simulink model "towing_project"  (Simulink 10.1)
settings: Solver=ode4  StartTime=0.0  StopTime=800  FixedStep=1  RelTol=1e-3  EnableMultiTasking=on
PreLoadFcn:
  | load('Initialization_data.mat');
undefined symbols (not defined in the file): D, D1, M, M1, Ma, Ma1, magnitude, p00, p10, p20, p30, p40
libraries: simulink x10, simulink_extras x4
(part 2 of 2)

== system towing_project/local DP1/Tug DP controller/[-inf inf] to [-pi pi]2 ==
  note: r
  note: x
  x [-inf inf] : Inport
  Constant : Constant  Value=2*pi
  Gain : Gain  Gain=pi  SaturateOnIntegerOverflow=on  OutDataTypeStr=Inherit: Same as input  ParamDataTypeStr=Inherit: Same as input
  Math Function : Math  Operator=rem  SignedPower=on  SaturateOnIntegerOverflow=on
  Saturation : Saturate  UpperLimit=1e10  LowerLimit=-1e10
  Sign : Signum
  Sum : Sum  Inputs=|+-  SaturateOnIntegerOverflow=on
  Sum1 : Sum  Inputs=|++  SaturateOnIntegerOverflow=on
  y [-pi pi] : Outport
  wires:
  Saturation/1 -> Sign/1, Sum1/1
  Sum/1 -> y [-pi pi]/1
  Math Function/1 -> Sum/1
  Constant/1 -> Math Function/2
  Sum1/1 -> Math Function/1
  Gain/1 -> Sum1/2, Sum/2
  Sign/1 -> Gain/1
  x [-inf inf]/1 -> Saturation/1

== system towing_project/local DP2/Tug/Coriolis and centripetal forces ==
  nu : Inport
  Mux : Mux  Inputs=3
  Selector1 : Selector  InputPortWidth=3  IndexOptions=Index vector (dialog)  Indices=[1 ]  OutputSizes=1
  Selector2 : Selector  InputPortWidth=3  IndexOptions=Index vector (dialog)  Indices=[2]  OutputSizes=1
  Selector3 : Selector  InputPortWidth=3  IndexOptions=Index vector (dialog)  Indices=[3]  OutputSizes=1
  Subsystem : Subsystem
  Subsystem1 : Subsystem
  Subsystem2 : Subsystem
  Output : Outport
  wires:
  nu/1 -> Selector1/1, Selector2/1, Selector3/1
  Selector2/1 -> Subsystem/1(v), Subsystem2/2(v)  "v"
  Selector3/1 -> Subsystem/2(r), Subsystem1/2(r), Subsystem2/3(r)  "r"
  Selector1/1 -> Subsystem1/1(u), Subsystem2/1(u)  "u"
  Subsystem/1(x direction) -> Mux/1
  Subsystem1/1(y direction) -> Mux/2
  Subsystem2/1(yaw direction) -> Mux/3
  Mux/1 -> Output/1

== system towing_project/local DP2/Tug/In Case of singularity ==
  input : Inport
  Compare To Constant : simulink/Logic and Bit Operations/Compare To Constant  relop=>=  const=1e8  OutDataTypeStr=boolean
  Stop Simulation : Stop
  output : Outport
  wires:
  input/1 -> output/1, Compare To Constant/1
  Compare To Constant/1 -> Stop Simulation/1

== system towing_project/local DP2/Tug/In Case of singularity1 ==
  input : Inport
  Compare To Constant : simulink/Logic and Bit Operations/Compare To Constant  relop=>=  const=1e10  OutDataTypeStr=boolean
  Stop Simulation : Stop
  output : Outport
  wires:
  input/1 -> output/1, Compare To Constant/1
  Compare To Constant/1 -> Stop Simulation/1

== system towing_project/local DP2/Tug/Rotation matrix in yaw ==
  psi : Inport
  nu : Inport  Port=2
  Fcn : Fcn  Expr=cos(u(1))*u(2)-sin(u(1))*u(3)
  Fcn1 : Fcn  Expr=sin(u(1))*u(2)+cos(u(1))*u(3)
  Fcn2 : Fcn  Expr=u(4)
  Mux : Mux  Inputs=2
  Mux1 : Mux  Inputs=3
  R*nu : Outport
  wires:
  Mux1/1 -> R*nu/1  "eta_dot"
  Mux/1 -> Fcn/1, Fcn1/1, Fcn2/1
  psi/1 -> Mux/1
  nu/1 -> Mux/2
  Fcn1/1 -> Mux1/2  "y_dot"
  Fcn/1 -> Mux1/1  "x_dot"
  Fcn2/1 -> Mux1/3  "psi_dot"

== system towing_project/local DP2/Tug/[-inf inf] to [-pi pi]1 ==
  note: x
  note: r
  x [-inf inf] : Inport
  Constant : Constant  Value=2*pi
  Gain : Gain  Gain=pi  SaturateOnIntegerOverflow=on  OutDataTypeStr=Inherit: Same as input  ParamDataTypeStr=Inherit: Same as input
  Math Function : Math  Operator=rem  SignedPower=on  SaturateOnIntegerOverflow=on
  Saturation : Saturate  UpperLimit=1e10  LowerLimit=-1e10
  Sign : Signum
  Sum : Sum  Inputs=|+-  SaturateOnIntegerOverflow=on
  Sum1 : Sum  Inputs=|++  SaturateOnIntegerOverflow=on
  y [-pi pi] : Outport
  wires:
  x [-inf inf]/1 -> Saturation/1
  Sign/1 -> Gain/1
  Gain/1 -> Sum/2, Sum1/2
  Sum1/1 -> Math Function/1
  Constant/1 -> Math Function/2
  Math Function/1 -> Sum/1
  Sum/1 -> y [-pi pi]/1
  Saturation/1 -> Sum1/1, Sign/1

== system towing_project/local DP2/Tug DP controller/Transposed rotation  matrix in yaw ==
  psi : Inport
  V : Inport  Port=2
  Mux : Mux  Inputs=2
  Mux1 : Mux  Inputs=3
  Row1 : Fcn  Expr=cos(u(1))*u(2)+sin(u(1))*u(3)
  Row2 : Fcn  Expr=-sin(u(1))*u(2)+cos(u(1))*u(3)
  Row3 : Fcn  Expr=u(4)
  Out1 : Outport
  wires:
  Mux/1 -> Row3/1, Row2/1, Row1/1
  Row1/1 -> Mux1/1
  Row2/1 -> Mux1/2
  Row3/1 -> Mux1/3
  Mux1/1 -> Out1/1
  psi/1 -> Mux/1
  V/1 -> Mux/2

== system towing_project/local DP2/Tug DP controller/[-inf inf] to [-pi pi]1 ==
  note: x
  note: r
  x [-inf inf] : Inport
  Constant : Constant  Value=2*pi
  Gain : Gain  Gain=pi  SaturateOnIntegerOverflow=on  OutDataTypeStr=Inherit: Same as input  ParamDataTypeStr=Inherit: Same as input
  Math Function : Math  Operator=rem  SignedPower=on  SaturateOnIntegerOverflow=on
  Saturation : Saturate  UpperLimit=1e10  LowerLimit=-1e10
  Sign : Signum
  Sum : Sum  Inputs=|+-  SaturateOnIntegerOverflow=on
  Sum1 : Sum  Inputs=|++  SaturateOnIntegerOverflow=on
  y [-pi pi] : Outport
  wires:
  x [-inf inf]/1 -> Saturation/1
  Sign/1 -> Gain/1
  Gain/1 -> Sum/2, Sum1/2
  Sum1/1 -> Math Function/1
  Constant/1 -> Math Function/2
  Math Function/1 -> Sum/1
  Sum/1 -> y [-pi pi]/1
  Saturation/1 -> Sum1/1, Sign/1

== system towing_project/local DP2/Tug DP controller/[-inf inf] to [-pi pi]2 ==
  note: r
  note: x
  x [-inf inf] : Inport
  Constant : Constant  Value=2*pi
  Gain : Gain  Gain=pi  SaturateOnIntegerOverflow=on  OutDataTypeStr=Inherit: Same as input  ParamDataTypeStr=Inherit: Same as input
  Math Function : Math  Operator=rem  SignedPower=on  SaturateOnIntegerOverflow=on
  Saturation : Saturate  UpperLimit=1e10  LowerLimit=-1e10
  Sign : Signum
  Sum : Sum  Inputs=|+-  SaturateOnIntegerOverflow=on
  Sum1 : Sum  Inputs=|++  SaturateOnIntegerOverflow=on
  y [-pi pi] : Outport
  wires:
  Saturation/1 -> Sign/1, Sum1/1
  Sum/1 -> y [-pi pi]/1
  Math Function/1 -> Sum/1
  Constant/1 -> Math Function/2
  Sum1/1 -> Math Function/1
  Gain/1 -> Sum1/2, Sum/2
  Sign/1 -> Gain/1
  x [-inf inf]/1 -> Saturation/1

== system towing_project/local DP3/Tug/Coriolis and centripetal forces ==
  nu : Inport
  Mux : Mux  Inputs=3
  Selector1 : Selector  InputPortWidth=3  IndexOptions=Index vector (dialog)  Indices=[1 ]  OutputSizes=1
  Selector2 : Selector  InputPortWidth=3  IndexOptions=Index vector (dialog)  Indices=[2]  OutputSizes=1
  Selector3 : Selector  InputPortWidth=3  IndexOptions=Index vector (dialog)  Indices=[3]  OutputSizes=1
  Subsystem : Subsystem
  Subsystem1 : Subsystem
  Subsystem2 : Subsystem
  Output : Outport
  wires:
  nu/1 -> Selector1/1, Selector2/1, Selector3/1
  Selector2/1 -> Subsystem/1(v), Subsystem2/2(v)  "v"
  Selector3/1 -> Subsystem/2(r), Subsystem1/2(r), Subsystem2/3(r)  "r"
  Selector1/1 -> Subsystem1/1(u), Subsystem2/1(u)  "u"
  Subsystem/1(x direction) -> Mux/1
  Subsystem1/1(y direction) -> Mux/2
  Subsystem2/1(yaw direction) -> Mux/3
  Mux/1 -> Output/1

== system towing_project/local DP3/Tug/In Case of singularity ==
  input : Inport
  Compare To Constant : simulink/Logic and Bit Operations/Compare To Constant  relop=>=  const=1e8  OutDataTypeStr=boolean
  Stop Simulation : Stop
  output : Outport
  wires:
  input/1 -> output/1, Compare To Constant/1
  Compare To Constant/1 -> Stop Simulation/1

== system towing_project/local DP3/Tug/In Case of singularity1 ==
  input : Inport
  Compare To Constant : simulink/Logic and Bit Operations/Compare To Constant  relop=>=  const=1e10  OutDataTypeStr=boolean
  Stop Simulation : Stop
  output : Outport
  wires:
  input/1 -> output/1, Compare To Constant/1
  Compare To Constant/1 -> Stop Simulation/1

== system towing_project/local DP3/Tug/Rotation matrix in yaw ==
  psi : Inport
  nu : Inport  Port=2
  Fcn : Fcn  Expr=cos(u(1))*u(2)-sin(u(1))*u(3)
  Fcn1 : Fcn  Expr=sin(u(1))*u(2)+cos(u(1))*u(3)
  Fcn2 : Fcn  Expr=u(4)
  Mux : Mux  Inputs=2
  Mux1 : Mux  Inputs=3
  R*nu : Outport
  wires:
  Mux1/1 -> R*nu/1  "eta_dot"
  Mux/1 -> Fcn/1, Fcn1/1, Fcn2/1
  psi/1 -> Mux/1
  nu/1 -> Mux/2
  Fcn1/1 -> Mux1/2  "y_dot"
  Fcn/1 -> Mux1/1  "x_dot"
  Fcn2/1 -> Mux1/3  "psi_dot"

== system towing_project/local DP3/Tug/[-inf inf] to [-pi pi]1 ==
  note: x
  note: r
  x [-inf inf] : Inport
  Constant : Constant  Value=2*pi
  Gain : Gain  Gain=pi  SaturateOnIntegerOverflow=on  OutDataTypeStr=Inherit: Same as input  ParamDataTypeStr=Inherit: Same as input
  Math Function : Math  Operator=rem  SignedPower=on  SaturateOnIntegerOverflow=on
  Saturation : Saturate  UpperLimit=1e10  LowerLimit=-1e10
  Sign : Signum
  Sum : Sum  Inputs=|+-  SaturateOnIntegerOverflow=on
  Sum1 : Sum  Inputs=|++  SaturateOnIntegerOverflow=on
  y [-pi pi] : Outport
  wires:
  x [-inf inf]/1 -> Saturation/1
  Sign/1 -> Gain/1
  Gain/1 -> Sum/2, Sum1/2
  Sum1/1 -> Math Function/1
  Constant/1 -> Math Function/2
  Math Function/1 -> Sum/1
  Sum/1 -> y [-pi pi]/1
  Saturation/1 -> Sum1/1, Sign/1

== system towing_project/local DP3/Tug DP controller/Transposed rotation  matrix in yaw ==
  psi : Inport
  V : Inport  Port=2
  Mux : Mux  Inputs=2
  Mux1 : Mux  Inputs=3
  Row1 : Fcn  Expr=cos(u(1))*u(2)+sin(u(1))*u(3)
  Row2 : Fcn  Expr=-sin(u(1))*u(2)+cos(u(1))*u(3)
  Row3 : Fcn  Expr=u(4)
  Out1 : Outport
  wires:
  Mux/1 -> Row3/1, Row2/1, Row1/1
  Row1/1 -> Mux1/1
  Row2/1 -> Mux1/2
  Row3/1 -> Mux1/3
  Mux1/1 -> Out1/1
  psi/1 -> Mux/1
  V/1 -> Mux/2

== system towing_project/local DP3/Tug DP controller/[-inf inf] to [-pi pi]1 ==
  note: x
  note: r
  x [-inf inf] : Inport
  Constant : Constant  Value=2*pi
  Gain : Gain  Gain=pi  SaturateOnIntegerOverflow=on  OutDataTypeStr=Inherit: Same as input  ParamDataTypeStr=Inherit: Same as input
  Math Function : Math  Operator=rem  SignedPower=on  SaturateOnIntegerOverflow=on
  Saturation : Saturate  UpperLimit=1e10  LowerLimit=-1e10
  Sign : Signum
  Sum : Sum  Inputs=|+-  SaturateOnIntegerOverflow=on
  Sum1 : Sum  Inputs=|++  SaturateOnIntegerOverflow=on
  y [-pi pi] : Outport
  wires:
  x [-inf inf]/1 -> Saturation/1
  Sign/1 -> Gain/1
  Gain/1 -> Sum/2, Sum1/2
  Sum1/1 -> Math Function/1
  Constant/1 -> Math Function/2
  Math Function/1 -> Sum/1
  Sum/1 -> y [-pi pi]/1
  Saturation/1 -> Sum1/1, Sign/1

== system towing_project/local DP3/Tug DP controller/[-inf inf] to [-pi pi]2 ==
  note: r
  note: x
  x [-inf inf] : Inport
  Constant : Constant  Value=2*pi
  Gain : Gain  Gain=pi  SaturateOnIntegerOverflow=on  OutDataTypeStr=Inherit: Same as input  ParamDataTypeStr=Inherit: Same as input
  Math Function : Math  Operator=rem  SignedPower=on  SaturateOnIntegerOverflow=on
  Saturation : Saturate  UpperLimit=1e10  LowerLimit=-1e10
  Sign : Signum
  Sum : Sum  Inputs=|+-  SaturateOnIntegerOverflow=on
  Sum1 : Sum  Inputs=|++  SaturateOnIntegerOverflow=on
  y [-pi pi] : Outport
  wires:
  Saturation/1 -> Sign/1, Sum1/1
  Sum/1 -> y [-pi pi]/1
  Math Function/1 -> Sum/1
  Constant/1 -> Math Function/2
  Sum1/1 -> Math Function/1
  Gain/1 -> Sum1/2, Sum/2
  Sign/1 -> Gain/1
  x [-inf inf]/1 -> Saturation/1

== system towing_project/local DP4/Tug/Coriolis and centripetal forces ==
  nu : Inport
  Mux : Mux  Inputs=3
  Selector1 : Selector  InputPortWidth=3  IndexOptions=Index vector (dialog)  Indices=[1 ]  OutputSizes=1
  Selector2 : Selector  InputPortWidth=3  IndexOptions=Index vector (dialog)  Indices=[2]  OutputSizes=1
  Selector3 : Selector  InputPortWidth=3  IndexOptions=Index vector (dialog)  Indices=[3]  OutputSizes=1
  Subsystem : Subsystem
  Subsystem1 : Subsystem
  Subsystem2 : Subsystem
  Output : Outport
  wires:
  nu/1 -> Selector1/1, Selector2/1, Selector3/1
  Selector2/1 -> Subsystem/1(v), Subsystem2/2(v)  "v"
  Selector3/1 -> Subsystem/2(r), Subsystem1/2(r), Subsystem2/3(r)  "r"
  Selector1/1 -> Subsystem1/1(u), Subsystem2/1(u)  "u"
  Subsystem/1(x direction) -> Mux/1
  Subsystem1/1(y direction) -> Mux/2
  Subsystem2/1(yaw direction) -> Mux/3
  Mux/1 -> Output/1

== system towing_project/local DP4/Tug/In Case of singularity ==
  input : Inport
  Compare To Constant : simulink/Logic and Bit Operations/Compare To Constant  relop=>=  const=1e8  OutDataTypeStr=boolean
  Stop Simulation : Stop
  output : Outport
  wires:
  input/1 -> output/1, Compare To Constant/1
  Compare To Constant/1 -> Stop Simulation/1

== system towing_project/local DP4/Tug/In Case of singularity1 ==
  input : Inport
  Compare To Constant : simulink/Logic and Bit Operations/Compare To Constant  relop=>=  const=1e10  OutDataTypeStr=boolean
  Stop Simulation : Stop
  output : Outport
  wires:
  input/1 -> output/1, Compare To Constant/1
  Compare To Constant/1 -> Stop Simulation/1

== system towing_project/local DP4/Tug/Rotation matrix in yaw ==
  psi : Inport
  nu : Inport  Port=2
  Fcn : Fcn  Expr=cos(u(1))*u(2)-sin(u(1))*u(3)
  Fcn1 : Fcn  Expr=sin(u(1))*u(2)+cos(u(1))*u(3)
  Fcn2 : Fcn  Expr=u(4)
  Mux : Mux  Inputs=2
  Mux1 : Mux  Inputs=3
  R*nu : Outport
  wires:
  Mux1/1 -> R*nu/1  "eta_dot"
  Mux/1 -> Fcn/1, Fcn1/1, Fcn2/1
  psi/1 -> Mux/1
  nu/1 -> Mux/2
  Fcn1/1 -> Mux1/2  "y_dot"
  Fcn/1 -> Mux1/1  "x_dot"
  Fcn2/1 -> Mux1/3  "psi_dot"

== system towing_project/local DP4/Tug/[-inf inf] to [-pi pi]1 ==
  note: x
  note: r
  x [-inf inf] : Inport
  Constant : Constant  Value=2*pi
  Gain : Gain  Gain=pi  SaturateOnIntegerOverflow=on  OutDataTypeStr=Inherit: Same as input  ParamDataTypeStr=Inherit: Same as input
  Math Function : Math  Operator=rem  SignedPower=on  SaturateOnIntegerOverflow=on
  Saturation : Saturate  UpperLimit=1e10  LowerLimit=-1e10
  Sign : Signum
  Sum : Sum  Inputs=|+-  SaturateOnIntegerOverflow=on
  Sum1 : Sum  Inputs=|++  SaturateOnIntegerOverflow=on
  y [-pi pi] : Outport
  wires:
  x [-inf inf]/1 -> Saturation/1
  Sign/1 -> Gain/1
  Gain/1 -> Sum/2, Sum1/2
  Sum1/1 -> Math Function/1
  Constant/1 -> Math Function/2
  Math Function/1 -> Sum/1
  Sum/1 -> y [-pi pi]/1
  Saturation/1 -> Sum1/1, Sign/1

== system towing_project/local DP4/Tug DP controller/Transposed rotation  matrix in yaw ==
  psi : Inport
  V : Inport  Port=2
  Mux : Mux  Inputs=2
  Mux1 : Mux  Inputs=3
  Row1 : Fcn  Expr=cos(u(1))*u(2)+sin(u(1))*u(3)
  Row2 : Fcn  Expr=-sin(u(1))*u(2)+cos(u(1))*u(3)
  Row3 : Fcn  Expr=u(4)
  Out1 : Outport
  wires:
  Mux/1 -> Row3/1, Row2/1, Row1/1
  Row1/1 -> Mux1/1
  Row2/1 -> Mux1/2
  Row3/1 -> Mux1/3
  Mux1/1 -> Out1/1
  psi/1 -> Mux/1
  V/1 -> Mux/2

== system towing_project/local DP4/Tug DP controller/[-inf inf] to [-pi pi]1 ==
  note: x
  note: r
  x [-inf inf] : Inport
  Constant : Constant  Value=2*pi
  Gain : Gain  Gain=pi  SaturateOnIntegerOverflow=on  OutDataTypeStr=Inherit: Same as input  ParamDataTypeStr=Inherit: Same as input
  Math Function : Math  Operator=rem  SignedPower=on  SaturateOnIntegerOverflow=on
  Saturation : Saturate  UpperLimit=1e10  LowerLimit=-1e10
  Sign : Signum
  Sum : Sum  Inputs=|+-  SaturateOnIntegerOverflow=on
  Sum1 : Sum  Inputs=|++  SaturateOnIntegerOverflow=on
  y [-pi pi] : Outport
  wires:
  x [-inf inf]/1 -> Saturation/1
  Sign/1 -> Gain/1
  Gain/1 -> Sum/2, Sum1/2
  Sum1/1 -> Math Function/1
  Constant/1 -> Math Function/2
  Math Function/1 -> Sum/1
  Sum/1 -> y [-pi pi]/1
  Saturation/1 -> Sum1/1, Sign/1

== system towing_project/local DP4/Tug DP controller/[-inf inf] to [-pi pi]2 ==
  note: r
  note: x
  x [-inf inf] : Inport
  Constant : Constant  Value=2*pi
  Gain : Gain  Gain=pi  SaturateOnIntegerOverflow=on  OutDataTypeStr=Inherit: Same as input  ParamDataTypeStr=Inherit: Same as input
  Math Function : Math  Operator=rem  SignedPower=on  SaturateOnIntegerOverflow=on
  Saturation : Saturate  UpperLimit=1e10  LowerLimit=-1e10
  Sign : Signum
  Sum : Sum  Inputs=|+-  SaturateOnIntegerOverflow=on
  Sum1 : Sum  Inputs=|++  SaturateOnIntegerOverflow=on
  y [-pi pi] : Outport
  wires:
  Saturation/1 -> Sign/1, Sum1/1
  Sum/1 -> y [-pi pi]/1
  Math Function/1 -> Sum/1
  Constant/1 -> Math Function/2
  Sum1/1 -> Math Function/1
  Gain/1 -> Sum1/2, Sum/2
  Sign/1 -> Gain/1
  x [-inf inf]/1 -> Saturation/1

== system towing_project/local DP1/Tug/Coriolis and centripetal forces/Subsystem ==
  v : Inport
  r : Inport  Port=2
  -a22 : Gain  Gain=-M1(2,2)-Ma1(2,2)  Multiplication=Matrix(K*u)  SaturateOnIntegerOverflow=on  OutDataTypeStr=Inherit: Same as input  ParamDataTypeStr=Inherit: Same as input
  -a26 : Gain  Gain=-M1(2,3)-Ma1(2,3)  Multiplication=Matrix(K*u)  SaturateOnIntegerOverflow=on  OutDataTypeStr=Inherit: Same as input  ParamDataTypeStr=Inherit: Same as input
  Add : Sum
  Math Function : Math  Operator=magnitude^2  SignedPower=on  SaturateOnIntegerOverflow=on
  Product : Product  RndMeth=Zero
  x direction : Outport
  wires:
  v/1 -> Product/1
  r/1 -> Product/2, Math Function/1
  Product/1 -> -a22/1
  Math Function/1 -> -a26/1
  -a22/1 -> Add/1
  -a26/1 -> Add/2
  Add/1 -> x direction/1

== system towing_project/local DP1/Tug/Coriolis and centripetal forces/Subsystem1 ==
  u : Inport
  r : Inport  Port=2
  Product : Product  RndMeth=Zero
  a11 : Gain  Gain=M1(1,1)+Ma1(1,1)  Multiplication=Matrix(K*u)  SaturateOnIntegerOverflow=on  OutDataTypeStr=Inherit: Same as input  ParamDataTypeStr=Inherit: Same as input
  y direction : Outport
  wires:
  Product/1 -> a11/1
  r/1 -> Product/2
  u/1 -> Product/1
  a11/1 -> y direction/1

== system towing_project/local DP1/Tug/Coriolis and centripetal forces/Subsystem2 ==
  u : Inport
  v : Inport  Port=2
  r : Inport  Port=3
  Add : Sum
  Add1 : Sum  Inputs=+-
  Product : Product  RndMeth=Zero
  Product1 : Product  RndMeth=Zero
  a11 : Gain  Gain=M1(1,1)+Ma1(1,1)  Multiplication=Matrix(K*u)  SaturateOnIntegerOverflow=on  OutDataTypeStr=Inherit: Same as input  ParamDataTypeStr=Inherit: Same as input
  a22 : Gain  Gain=M1(2,2)+Ma1(2,2)  Multiplication=Matrix(K*u)  SaturateOnIntegerOverflow=on  OutDataTypeStr=Inherit: Same as input  ParamDataTypeStr=Inherit: Same as input
  a62 : Gain  Gain=M1(3,2)+Ma1(3,2)  Multiplication=Matrix(K*u)  SaturateOnIntegerOverflow=on  OutDataTypeStr=Inherit: Same as input  ParamDataTypeStr=Inherit: Same as input
  yaw direction : Outport
  wires:
  u/1 -> Product/1, Product1/1
  r/1 -> Product/2
  Product/1 -> a62/1
  v/1 -> Product1/2
  Product1/1 -> a22/1, a11/1
  a22/1 -> Add1/1
  a11/1 -> Add1/2
  Add1/1 -> Add/2
  a62/1 -> Add/1
  Add/1 -> yaw direction/1

== system towing_project/local DP2/Tug/Coriolis and centripetal forces/Subsystem ==
  v : Inport
  r : Inport  Port=2
  -a22 : Gain  Gain=-M1(2,2)-Ma1(2,2)  Multiplication=Matrix(K*u)  SaturateOnIntegerOverflow=on  OutDataTypeStr=Inherit: Same as input  ParamDataTypeStr=Inherit: Same as input
  -a26 : Gain  Gain=-M1(2,3)-Ma1(2,3)  Multiplication=Matrix(K*u)  SaturateOnIntegerOverflow=on  OutDataTypeStr=Inherit: Same as input  ParamDataTypeStr=Inherit: Same as input
  Add : Sum
  Math Function : Math  Operator=magnitude^2  SignedPower=on  SaturateOnIntegerOverflow=on
  Product : Product  RndMeth=Zero
  x direction : Outport
  wires:
  v/1 -> Product/1
  r/1 -> Product/2, Math Function/1
  Product/1 -> -a22/1
  Math Function/1 -> -a26/1
  -a22/1 -> Add/1
  -a26/1 -> Add/2
  Add/1 -> x direction/1

== system towing_project/local DP2/Tug/Coriolis and centripetal forces/Subsystem1 ==
  u : Inport
  r : Inport  Port=2
  Product : Product  RndMeth=Zero
  a11 : Gain  Gain=M1(1,1)+Ma1(1,1)  Multiplication=Matrix(K*u)  SaturateOnIntegerOverflow=on  OutDataTypeStr=Inherit: Same as input  ParamDataTypeStr=Inherit: Same as input
  y direction : Outport
  wires:
  Product/1 -> a11/1
  r/1 -> Product/2
  u/1 -> Product/1
  a11/1 -> y direction/1

== system towing_project/local DP2/Tug/Coriolis and centripetal forces/Subsystem2 ==
  u : Inport
  v : Inport  Port=2
  r : Inport  Port=3
  Add : Sum
  Add1 : Sum  Inputs=+-
  Product : Product  RndMeth=Zero
  Product1 : Product  RndMeth=Zero
  a11 : Gain  Gain=M1(1,1)+Ma1(1,1)  Multiplication=Matrix(K*u)  SaturateOnIntegerOverflow=on  OutDataTypeStr=Inherit: Same as input  ParamDataTypeStr=Inherit: Same as input
  a22 : Gain  Gain=M1(2,2)+Ma1(2,2)  Multiplication=Matrix(K*u)  SaturateOnIntegerOverflow=on  OutDataTypeStr=Inherit: Same as input  ParamDataTypeStr=Inherit: Same as input
  a62 : Gain  Gain=M1(3,2)+Ma1(3,2)  Multiplication=Matrix(K*u)  SaturateOnIntegerOverflow=on  OutDataTypeStr=Inherit: Same as input  ParamDataTypeStr=Inherit: Same as input
  yaw direction : Outport
  wires:
  u/1 -> Product/1, Product1/1
  r/1 -> Product/2
  Product/1 -> a62/1
  v/1 -> Product1/2
  Product1/1 -> a22/1, a11/1
  a22/1 -> Add1/1
  a11/1 -> Add1/2
  Add1/1 -> Add/2
  a62/1 -> Add/1
  Add/1 -> yaw direction/1

== system towing_project/local DP3/Tug/Coriolis and centripetal forces/Subsystem ==
  v : Inport
  r : Inport  Port=2
  -a22 : Gain  Gain=-M1(2,2)-Ma1(2,2)  Multiplication=Matrix(K*u)  SaturateOnIntegerOverflow=on  OutDataTypeStr=Inherit: Same as input  ParamDataTypeStr=Inherit: Same as input
  -a26 : Gain  Gain=-M1(2,3)-Ma1(2,3)  Multiplication=Matrix(K*u)  SaturateOnIntegerOverflow=on  OutDataTypeStr=Inherit: Same as input  ParamDataTypeStr=Inherit: Same as input
  Add : Sum
  Math Function : Math  Operator=magnitude^2  SignedPower=on  SaturateOnIntegerOverflow=on
  Product : Product  RndMeth=Zero
  x direction : Outport
  wires:
  v/1 -> Product/1
  r/1 -> Product/2, Math Function/1
  Product/1 -> -a22/1
  Math Function/1 -> -a26/1
  -a22/1 -> Add/1
  -a26/1 -> Add/2
  Add/1 -> x direction/1

== system towing_project/local DP3/Tug/Coriolis and centripetal forces/Subsystem1 ==
  u : Inport
  r : Inport  Port=2
  Product : Product  RndMeth=Zero
  a11 : Gain  Gain=M1(1,1)+Ma1(1,1)  Multiplication=Matrix(K*u)  SaturateOnIntegerOverflow=on  OutDataTypeStr=Inherit: Same as input  ParamDataTypeStr=Inherit: Same as input
  y direction : Outport
  wires:
  Product/1 -> a11/1
  r/1 -> Product/2
  u/1 -> Product/1
  a11/1 -> y direction/1

== system towing_project/local DP3/Tug/Coriolis and centripetal forces/Subsystem2 ==
  u : Inport
  v : Inport  Port=2
  r : Inport  Port=3
  Add : Sum
  Add1 : Sum  Inputs=+-
  Product : Product  RndMeth=Zero
  Product1 : Product  RndMeth=Zero
  a11 : Gain  Gain=M1(1,1)+Ma1(1,1)  Multiplication=Matrix(K*u)  SaturateOnIntegerOverflow=on  OutDataTypeStr=Inherit: Same as input  ParamDataTypeStr=Inherit: Same as input
  a22 : Gain  Gain=M1(2,2)+Ma1(2,2)  Multiplication=Matrix(K*u)  SaturateOnIntegerOverflow=on  OutDataTypeStr=Inherit: Same as input  ParamDataTypeStr=Inherit: Same as input
  a62 : Gain  Gain=M1(3,2)+Ma1(3,2)  Multiplication=Matrix(K*u)  SaturateOnIntegerOverflow=on  OutDataTypeStr=Inherit: Same as input  ParamDataTypeStr=Inherit: Same as input
  yaw direction : Outport
  wires:
  u/1 -> Product/1, Product1/1
  r/1 -> Product/2
  Product/1 -> a62/1
  v/1 -> Product1/2
  Product1/1 -> a22/1, a11/1
  a22/1 -> Add1/1
  a11/1 -> Add1/2
  Add1/1 -> Add/2
  a62/1 -> Add/1
  Add/1 -> yaw direction/1

== system towing_project/local DP4/Tug/Coriolis and centripetal forces/Subsystem ==
  v : Inport
  r : Inport  Port=2
  -a22 : Gain  Gain=-M1(2,2)-Ma1(2,2)  Multiplication=Matrix(K*u)  SaturateOnIntegerOverflow=on  OutDataTypeStr=Inherit: Same as input  ParamDataTypeStr=Inherit: Same as input
  -a26 : Gain  Gain=-M1(2,3)-Ma1(2,3)  Multiplication=Matrix(K*u)  SaturateOnIntegerOverflow=on  OutDataTypeStr=Inherit: Same as input  ParamDataTypeStr=Inherit: Same as input
  Add : Sum
  Math Function : Math  Operator=magnitude^2  SignedPower=on  SaturateOnIntegerOverflow=on
  Product : Product  RndMeth=Zero
  x direction : Outport
  wires:
  v/1 -> Product/1
  r/1 -> Product/2, Math Function/1
  Product/1 -> -a22/1
  Math Function/1 -> -a26/1
  -a22/1 -> Add/1
  -a26/1 -> Add/2
  Add/1 -> x direction/1

== system towing_project/local DP4/Tug/Coriolis and centripetal forces/Subsystem1 ==
  u : Inport
  r : Inport  Port=2
  Product : Product  RndMeth=Zero
  a11 : Gain  Gain=M1(1,1)+Ma1(1,1)  Multiplication=Matrix(K*u)  SaturateOnIntegerOverflow=on  OutDataTypeStr=Inherit: Same as input  ParamDataTypeStr=Inherit: Same as input
  y direction : Outport
  wires:
  Product/1 -> a11/1
  r/1 -> Product/2
  u/1 -> Product/1
  a11/1 -> y direction/1

== system towing_project/local DP4/Tug/Coriolis and centripetal forces/Subsystem2 ==
  u : Inport
  v : Inport  Port=2
  r : Inport  Port=3
  Add : Sum
  Add1 : Sum  Inputs=+-
  Product : Product  RndMeth=Zero
  Product1 : Product  RndMeth=Zero
  a11 : Gain  Gain=M1(1,1)+Ma1(1,1)  Multiplication=Matrix(K*u)  SaturateOnIntegerOverflow=on  OutDataTypeStr=Inherit: Same as input  ParamDataTypeStr=Inherit: Same as input
  a22 : Gain  Gain=M1(2,2)+Ma1(2,2)  Multiplication=Matrix(K*u)  SaturateOnIntegerOverflow=on  OutDataTypeStr=Inherit: Same as input  ParamDataTypeStr=Inherit: Same as input
  a62 : Gain  Gain=M1(3,2)+Ma1(3,2)  Multiplication=Matrix(K*u)  SaturateOnIntegerOverflow=on  OutDataTypeStr=Inherit: Same as input  ParamDataTypeStr=Inherit: Same as input
  yaw direction : Outport
  wires:
  u/1 -> Product/1, Product1/1
  r/1 -> Product/2
  Product/1 -> a62/1
  v/1 -> Product1/2
  Product1/1 -> a22/1, a11/1
  a22/1 -> Add1/1
  a11/1 -> Add1/2
  Add1/1 -> Add/2
  a62/1 -> Add/1
  Add/1 -> yaw direction/1

== matlab function Cable Force ==
  data: tau0 output double; state input double; tau1 output double; tau2 output double; tau3 output double; tau4 output double
function [tau0, tau1, tau2, tau3, tau4] = cable_force(state)

%% 锚链
    Kc = 6e4;
    L10 = 459;
    L20 = 459;
    L30 = 459;
    L40 = 459;
    
    x0 = [-75, 75, 75, -75, -75];
    y0 = [50, 50, -50, -50, 50];
    x1 = [-16, 12, 16, 12, -16, -16];
    y1 = [6, 6, 0, -6, -6, 6];
    x2 = [-16, 12, 16, 12, -16, -16];
    y2 = [6, 6, 0, -6, -6, 6];
    
    p0 = state(1 : 3);
    p1 = state(4 : 6);
    p2 = state(10 : 12);
    p3 = state(16 : 18);
    p4 = state(22 : 24);
    
    
    % 角度转化成弧度
    p0(3) = p0(3) * pi / 180;
    p1(3) = p1(3) * pi / 180;
    p2(3) = p2(3) * pi / 180;
    p3(3) = p3(3) * pi / 180;
    p4(3) = p4(3) * pi / 180;
    
    % 缆绳起始点坐标（全局坐标系下）
    pc1_start = local_to_global([x0(2); y0(2)], p0);
    pc1_end = local_to_global([(x1(1)+x1(5))/2; (y1(1)+y1(5))/2], p1);
    pc2_start = local_to_global([x0(3); y0(3)], p0);
    pc2_end = local_to_global([(x2(1)+x2(5))/2; (y2(1)+y2(5))/2], p2);
    pc3_start = local_to_global([x0(4); y0(4)], p0);
    pc3_end = local_to_global([(x1(1)+x1(5))/2; (y1(1)+y1(5))/2], p3);
    pc4_start = local_to_global([x0(5); y0(5)], p0);
    pc4_end = local_to_global([(x2(1)+x2(5))/2; (y2(1)+y2(5))/2], p4);
    
    % 缆绳长度
    Lc1 = sqrt((pc1_start(1) - pc1_end(1)) ^ 2 + (pc1_start(2) - pc1_end(2)) ^ 2 );
    Lc2 = sqrt((pc2_start(1) - pc2_end(1)) ^ 2 + (pc2_start(2) - pc2_end(2)) ^ 2 );
    Lc3 = sqrt((pc3_start(1) - pc3_end(1)) ^ 2 + (pc3_start(2) - pc3_end(2)) ^ 2 );
    Lc4 = sqrt((pc4_start(1) - pc4_end(1)) ^ 2 + (pc4_start(2) - pc4_end(2)) ^ 2 );
    
    % 缆绳张力
    % 缆绳张力
    if (Lc1 >= L10)
        fc1 = Kc * (Lc1 - L10);
    else
        fc1 = 0;
    end
    
    if (Lc2 >= L20)
        fc2 = Kc * (Lc2 - L20);
    else
        fc2 = 0;
    end
    
    if (Lc3 >= L30)
        fc3 = Kc * (Lc3 - L30);
    else
        fc3 = 0;
    end
    
    if (Lc4 >= L40)
        fc4 = Kc * (Lc4 - L40);
    else
        fc4 = 0;
    end
    
    % 缆绳角度(全局坐标系）
    alpha1 = atan2( -(pc1_start(2) - pc1_end(2)), -(pc1_start(1) - pc1_end(1)) );
    alpha2 = atan2( -(pc2_start(2) - pc2_end(2)), -(pc2_start(1) - pc2_end(1)) );
    alpha3 = atan2( -(pc3_start(2) - pc3_end(2)), -(pc3_start(1) - pc3_end(1)) );
    alpha4 = atan2( -(pc4_start(2) - pc4_end(2)), -(pc4_start(1) - pc4_end(1)) );
    
    % 缆绳相对母船的角度（母船坐标系下）
    belta1 = alpha1 - p0(3);
    belta2 = alpha2 - p0(3);
    belta3 = alpha3 - p0(3);
    belta4 = alpha4 - p0(3);
    
    % 将角度转化为（-pi, pi)
    belta1 = transfer_deg(belta1);
    belta2 = transfer_deg(belta2);
    belta3 = transfer_deg(belta3);
    belta4 = transfer_deg(belta4);
    
    % 母船局部坐标系下
    tau10 = fc1 * [ cos(belta1),  sin(belta1), -y0(2) * cos(belta1) + x0(2) * sin(belta1) ]'
    tau20 = fc2 * [ cos(belta2),  sin(belta2), -y0(3) * cos(belta2) + x0(3) * sin(belta2) ]'
    tau30 = fc3 * [ cos(belta3),  sin(belta3), -y0(4) * cos(belta3) + x0(4) * sin(belta3) ]'
    tau40 = fc4 * [ cos(belta4),  sin(belta4), -y0(5) * cos(belta4) + x0(5) * sin(belta4) ]'
    tau0 = tau10 + tau20 + tau30 + tau40;
    
    
    % 缆绳力相对拖轮的角度（拖轮局部坐标系下）
    gama1 = pi - (p1(3) - alpha1);  gama1 = transfer_deg(gama1);
    gama2 = pi - (p2(3) - alpha2);  gama2 = transfer_deg(gama2);
    gama3 = pi - (p3(3) - alpha3);  gama3 = transfer_deg(gama3);
    gama4 = pi - (p4(3) - alpha4);  gama4 = transfer_deg(gama4);
    
    % 缆绳作用在拖轮上的力，拖轮局部坐标系下
    tau1 = fc1 * [cos(gama1), sin(gama1), (x1(1)+x1(5))/2 * sin(gama1) - (y1(1)+y1(5))/2 * cos(gama1)]'
    tau2 = fc2 * [cos(gama2), sin(gama2), (x1(1)+x1(5))/2 * sin(gama2) - (y1(1)+y1(5))/2 * cos(gama2)]'
    tau3 = fc3 * [cos(gama3), sin(gama3), (x1(1)+x1(5))/2 * sin(gama3) - (y1(1)+y1(5))/2 * cos(gama3)]'
    tau4 = fc4 * [cos(gama4), sin(gama4), (x1(1)+x1(5))/2 * sin(gama4) - (y1(1)+y1(5))/2 * cos(gama4)]'
end


%% 寻找锚链连接点(大地坐标系下）
function pc_g = local_to_global(pc_l, p0)
    fai = p0(3);
    R = [cos(fai), -sin(fai);
        sin(fai), cos(fai)];
    pc_g = R * pc_l + p0(1:2);
    
end

%% 旋转矩阵
function [R2, R3] = rotate_matrix(p)

    fai = p(3);
    R2  = [cos(fai), -sin(fai);
            sin(fai), cos(fai)];
    
    R3 = [cos(fai), -sin(fai), 0;
        sin(fai), cos(fai), 0;
        0, 0, 1];
end

%% 将角度转化为（-pi, pi)
function y = transfer_deg(x)
    y = -sign(x) * pi + rem((x + sign(x) * pi), 2 * pi);
end

== matlab function Consensus Control ==
  data: p0 input double; pd1 output double; v0 input double; state input double; pd2 output double; pd3 output double; pd4 output double
% function [pd1, pd2] = consensus_guidance(p0, v0, p1, v1, p2, v2)
function [pd1, pd2, pd3, pd4] = consensus_guidance(p0, v0, state)
% 默认输入和输出的单位为角度
% % p0, v0的角度单位都是弧度
% p(全局坐标系）， v(局部坐标系）
% dot_p (全局坐标系）
% clear all; clc;
% p1 = [397, 237, 31]';
% p2 = [397, -237, -31]';
% p0 = [1, 0, 0]';
% v0 = zeros(3, 1);
% v1 = zeros(3, 1);
% v2 = zeros(3, 1);

p1 = state(1:3);
v1 = state(4:6);
p2 = state(7:9);
v2 = state(10:12);
p3 = state(13 : 15);
v3 = state(16 : 18);
p4 = state(19 :21);
v4 = state(22 : 24);

% 需要声明lqr函数为外部函数，否则simulink会编译报错
coder.extrinsic('lqr'); 

pd1 = zeros(3, 1);
pd2 = zeros(3, 1);
pd3 = zeros(3, 1);
pd4 = zeros(3, 1);

% 角度单位转化成弧度
deg_to_rad = pi / 180;
p0(3) = p0(3) * deg_to_rad;
p1(3) = p1(3) * deg_to_rad;
p2(3) = p2(3) * deg_to_rad;
p3(3) = p3(3) * deg_to_rad;
p4(3) = p4(3) * deg_to_rad;

dotP0 = v0; % 输入的v0是在大地坐标系下的   
dotP0(3) = dotP0(3) * deg_to_rad;

% % 将角度转化为（-pi, pi)
% p0(3) = transfer_deg(p0(3));
% p1(3) = transfer_deg(p1(3));
% p2(3) = transfer_deg(p2(3));

% dotP0 = V_to_dotP(p0, v0);
dotP1 = V_to_dotP(p1, v1);
dotP2 = V_to_dotP(p2, v2);
dotP3 = V_to_dotP(p3, v3);
dotP4 = V_to_dotP(p4, v4);

% 定义状态变量
x0 = [p0; dotP0];
x1 = [p1; dotP1];
x2 = [p2; dotP2];
x3 = [p3; dotP3];
x4 = [p4; dotP4];

%% 编队的相对位置,这个是在局部坐标系下的，需要转化为大地坐标系下
deta10 = [397, 237, 31 * deg_to_rad, 0, 0, 0]';
deta20 = [397, -237, -31 * deg_to_rad, 0, 0, 0]';
deta30 = [-397, -237, -149 * deg_to_rad, 0, 0, 0]';
deta40 = [-397, 237, 149 * deg_to_rad, 0, 0, 0]';

deta12 = deta10 - deta20;   deta21 = -deta12;
deta14 = deta10 - deta40;   deta41 = -deta14;
deta23 = deta20 - deta30;   deta32 = -deta23;
deta34 = deta30 - deta40;   deta43 = -deta34;


fai0 = p0(3);   fai1 = p1(3);   fai2 = p2(3);
fai3 = p3(3);   fai4 = p4(3);

%拖船到母船的距离
Lc1 = sqrt(deta10(1)^2 + deta10(2)^2);
Lc2 = sqrt(deta20(1)^2 + deta20(2)^2);
Lc3 = sqrt(deta30(1)^2 + deta30(2)^2);
Lc4 = sqrt(deta40(1)^2 + deta40(2)^2);

deta10(1:2) = [cos(fai0), -sin(fai0); sin(fai0), cos(fai0)] * deta10(1:2);
deta20(1:2) = [cos(fai0), -sin(fai0); sin(fai0), cos(fai0)] * deta20(1:2);
deta30(1:2) = [cos(fai0), -sin(fai0); sin(fai0), cos(fai0)] * deta30(1:2);
deta40(1:2) = [cos(fai0), -sin(fai0); sin(fai0), cos(fai0)] * deta40(1:2);

deta12 = deta10 - deta20;   deta21 = -deta12;
deta14 = deta10 - deta40;   deta41 = -deta14;
deta23 = deta20 - deta30;   deta32 = -deta23;
deta34 = deta30 - deta40;   deta43 = -deta34;
% deta12 = deta10 - deta20;
% deta21 = - deta12;



% 先假定aij = 1, gi = 1;， 需要加上相对位置
e1 = x2 - x1 - deta21 + x4 - x1 - deta41 + x0 - x1 + deta10;
e2 = x1 - x2 - deta12 + x3 - x2 - deta32 + x0 - x2 + deta20;
e3 = x2 - x3 - deta23 + x4 - x3 - deta43 + x0 - x3 + deta30;
e4 = x1 - x4 - deta14 + x3 - x4 - deta34 + x0 - x4 + deta40;

e1(3) = transfer_deg(e1(3));
e2(3) = transfer_deg(e2(3));
e3(3) = transfer_deg(e3(3));
e4(3) = transfer_deg(e4(3));

%% 定义状态反馈方程的系数，求解raccati方程
wn = 0.05; 
cd = 0.7;

A1 = -2 * cd * wn * eye(3);
A0 = -wn^2 * eye(3);
B1 = -A0;

A = [zeros(3, 3), eye(3); A0, A1];
B = [zeros(3, 3); B1];

% Q = diag([0.01, 0.01, 4e-8, 100, 100, 4e-4]);
% R = diag([0.01, 0.01, 4e-8]);
Q = 4 * eye(6);
R = 1 * eye(3);
N = [];
[K, S, e] = lqr(A, B, Q, R, N);

K;
u1 = K * e1;
u2 = K * e2;
u3 = K * e3;
u4 = K * e4;

pd1 = u1; 
pd2 = u2;
pd3 = u3; 
pd4 = u4;

pd1 = pd1 + p1;
pd2 = pd2 + p2;
pd3 = pd3 + p3;
pd4 = pd4 + p4;

pd1(3) = transfer_deg(pd1(3));
pd2(3) = transfer_deg(pd2(3));
pd3(3) = transfer_deg(pd3(3));
pd4(3) = transfer_deg(pd4(3));


%% 函数输入输出都是角度
pd1(3) = pd1(3) / 3.14 * 180;
pd2(3) = pd2(3) / 3.14 * 180;
pd3(3) = pd3(3) / 3.14 * 180;
pd4(3) = pd4(3) / 3.14 * 180;

end







%% 旋转矩阵
function R = RotationMatrix(p)
fai = p(3);
R = zeros(3, 3);
R = [cos(fai), -sin(fai), 0;
    sin(fai), cos(fai), 0;
    0, 0, 1];
end

%% 将速度转换成全局坐标系中，即p的微分
function dot_P = V_to_dotP(p, v)
R = zeros(3, 3);
R = RotationMatrix(p);
dot_P = R * v;

end

%% 将角度转化为（-pi, pi)
function y = transfer_deg(x)
    y = -sign(x) * pi + rem((x + sign(x) * pi), 2 * pi);
end
